simulink model "PID_Sim"  (R2016b)
settings: Solver=VariableStepAuto  StartTime=0.0  StopTime=100  MaxStep=0.01  RelTol=1e-4  EnableMultiTasking=on
settings Model: Creator=Malte  LastModifiedBy=Malte
settings DataIOCC: LimitDataPoints=on  SaveOutput=off  SaveTime=off
settings OptimizationCC: ExpressionDepthLimit=2147483647  LifeSpan=1
settings DebuggingCC: UnderspecifiedInitializationDetection=Classic  MergeDetectMultiDrivingBlocksExec=none  FcnCallInpInsideContextMsg=warning  AllowSymbolicDim=off  StateNameClashWarn=warning  SFUnexpectedBacktrackingDiag=warning  SFNoUnconditionalDefaultTransitionDiag=warning  SFExecutionAtInitializationDiag=none
settings GRTTargetCC: TargetLangStandard=C89/C90 (ANSI)  GeneratePreprocessorConditionals=Disable all  CombineOutputUpdateFcns=off  GRTInterface=on

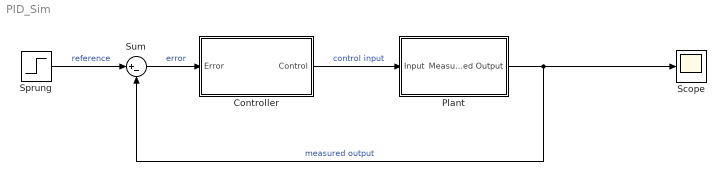
== system PID_Sim ==
  Controller : Subsystem
  Plant : Subsystem
  Scope : Scope
  Sprung : Step  SampleTime=0
  Sum : Sum  Inputs=|+-
  wires:
  Sprung/1 -> Sum/1  "reference"
  Plant/1(Measured Output) -> Sum/2, Scope/1  "measured output"
  Sum/1 -> Controller/1(Error)  "error"
  Controller/1(Control) -> Plant/1(Input)  "control input"

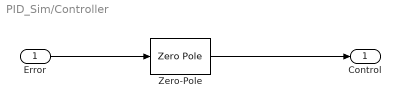
== system PID_Sim/Controller ==
  Error : Inport
  Zero-Pole : ZeroPole  Zeros=[-0.5]  Poles=[-1 -10]  Gain=[23]
  Control : Outport
  wires:
  Error/1 -> Zero-Pole/1
  Zero-Pole/1 -> Control/1

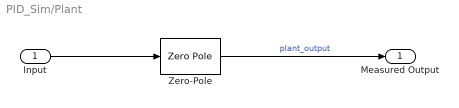
== system PID_Sim/Plant ==
  Input : Inport
  Zero-Pole : ZeroPole  Zeros=[]  Poles=[1 -1]
  Measured Output : Outport
  wires:
  Input/1 -> Zero-Pole/1
  Zero-Pole/1 -> Measured Output/1  "plant_output"
